simulink model "example_Hydraulic_HouseHeatingSystem"  (R2016b)
settings: Solver=ode23tb  StartTime=0.0  StopTime=2*24*3600  MaxStep=3600  RelTol=1e-3  EnableMultiTasking=on
undefined symbols (not defined in the file): path_carnot
libraries: carnot x12
settings Model: Creator=drhf  LastModifiedBy=drhf
settings DataIOCC: LimitDataPoints=on  SaveFormat=Array  SignalLoggingSaveFormat=ModelDataLogs
settings OptimizationCC: ExpressionDepthLimit=2147483647  LifeSpan=inf
settings DebuggingCC: UnderspecifiedInitializationDetection=Classic  MergeDetectMultiDrivingBlocksExec=none  SolverPrmCheckMsg=warning  FcnCallInpInsideContextMsg=warning  StateNameClashWarn=warning  SFUnexpectedBacktrackingDiag=warning  SFNoUnconditionalDefaultTransitionDiag=warning  SFExecutionAtInitializationDiag=none
settings HardwareCC: ProdBitPerPointer=32  ProdBitPerSizeT=32  ProdBitPerPtrDiffT=32  ProdLargestAtomicFloat=None  ProdIntDivRoundTo=Undefined  ProdEndianess=Unspecified  ProdWordSize=32  ProdHWDeviceType=32-bit Generic
settings ModelReferenceCC: PropagateSignalLabelsOutOfModel=off
settings GRTTargetCC: TargetLangStandard=C89/C90 (ANSI)  GeneratePreprocessorConditionals=Disable all  CombineOutputUpdateFcns=off  GRTInterface=on
settings ConfigComp: CovMetricSettings=dw  CovHtmlReporting=on  CovSaveCumulativeToWorkspaceVar=on  CovSaveSingleToWorkspaceVar=on  CovExternalEMLEnable=off

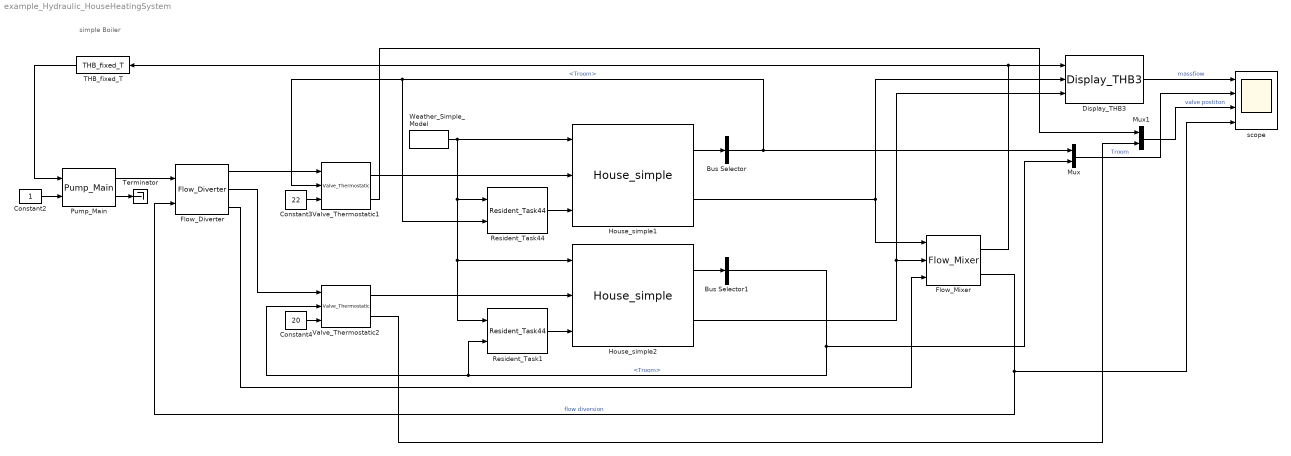
== system example_Hydraulic_HouseHeatingSystem ==
  note: simple Boiler
  Bus Selector : BusSelector  OutputSignals=Troom
  Bus Selector1 : BusSelector  OutputSignals=Troom
  Constant2 : Constant
  Constant3 : Constant  Value=22
  Constant4 : Constant  Value=20
  Display_THB3 : carnot/Outputs/Display_THB3  t=off  m=on  p=off  id=off  mix=off  d=off
  Flow_Diverter : carnot/Hydraulics/Flow_Diverter
  Flow_Mixer : carnot/Hydraulics/Flow_Mixer  t=1
  House_simple1 : carnot/Load/Houses/House_simple  tini=20  dtroom=inf  Tmeaninside=23.8  deltathetai=3.8  Tmeanoutside=11  deltathetae=9.3  tshift=319*3600  PathName=fullfile(path_carnot('libsl'), 'Load', 'Houses', 'House_simple', 'parameter_set')  FileName='SimpleHouse_Room40m2.mat'  userPath=off  userParam=off  Ahabit=40  Hroom=2.5  slabwidth=10  slablength=7  dwall=0.4  UAwall=100  capa=500000  utot=0.183  gammat=0  cond_ground=2  cp_ground=800  rho_ground=2500  Awindow=[12 4 3 4]  AziWin=[0 90 -180 -90]  Uwindow=[2 2 2 2]  Gwindow=[0.5 0.5 0.5 0.5]  alpha=10  H=1.2  W=1  Nwin=4  Ventilationrate=0.4  Heatrecovery=0  pnom=10000  dtnom=49.83  expo=1.3  mcap=10*4812  lin=100  qua=100
  House_simple2 : carnot/Load/Houses/House_simple  tini=20  dtroom=inf  Tmeaninside=23.8  deltathetai=3.8  Tmeanoutside=11  deltathetae=9.3  tshift=319*3600  PathName=fullfile(path_carnot('libsl'), 'Load', 'Houses', 'House_simple', 'parameter_set')  FileName='SimpleHouse_Room40m2.mat'  userPath=off  userParam=off  Ahabit=40  Hroom=2.5  slabwidth=10  slablength=7  dwall=0.4  UAwall=100  capa=500000  utot=0.183  gammat=0  cond_ground=2  cp_ground=800  rho_ground=2500  Awindow=[12 4 3 4]  AziWin=[0 90 -180 -90]  Uwindow=[2 2 2 2]  Gwindow=[0.5 0.5 0.5 0.5]  alpha=10  H=1.2  W=1  Nwin=4  Ventilationrate=0.4  Heatrecovery=0  pnom=10000  dtnom=49.83  expo=1.3  mcap=10*4812  lin=100  qua=100
  Mux : Mux  Inputs=2
  Mux1 : Mux  Inputs=2
  Pump_Main : carnot/Hydraulics/Pump_Main  Tini=20  p0=3e5  IDpreset=pressure drop  fluid=Water  mix=0  mix2=0  mix3=0  t1=1  PathName=fullfile(path_carnot('libsl'), 'Hydraulics', 'Pump_Main', 'parameter_set')  FileName='Pump6m.mat'  userPath=off  userParam=off  a0=60000  a1=-43200  a2=0  dia=0.025  UA=1  mcp=4182  e0=50  e1=28.8  e2=-10.368
  Resident_Task1 : carnot/Load/Houses/Resident_Task44  period=24*3600  rep_seq_te=[0 1 6 7 8 9 11 12 13 18 19 20 22 23]*3600  rep_seq_de=[1 5 1 1 1 2 1 1 4 2 1 2 1 1]*3600  rep_seq_ye=[105 55 392.5 457.5 420 55 250 55 120 170 615 420 442.5 355]/3  rep_seq_to=[0 6 7 8 9 11 12 13 14 15 17 18 20 21 22]*3600  rep_seq_do=[6 1 1 1 2 1 1 1 1 2 1 2 1 1 2]*3600  rep_seq_yo=[4 2 3 2 0 1 3 2 1 0 1 2 4 3 4]*60/2  Topen=24  Tclose=23  TrAboveTa=2  TaTooCold=12  timeFIR=24  TaIni=12  starttime=8  stoptime=22  TroomShadeOn=23.8  TroomShadeOff=22.8  SolarShadeOn=300  SolarShadeOff=200  max_shade=1  CalcAirComp=off  mdotCO2=0  mdotH2O=0  mdotVOC=0
  Resident_Task44 : carnot/Load/Houses/Resident_Task44  period=24*3600  rep_seq_te=[0 1 6 7 8 9 11 12 13 18 19 20 22 23]*3600  rep_seq_de=[1 5 1 1 1 2 1 1 4 2 1 2 1 1]*3600  rep_seq_ye=[105 55 392.5 457.5 420 55 250 55 120 170 615 420 442.5 355]/3  rep_seq_to=[0 6 7 8 9 11 12 13 14 15 17 18 20 21 22]*3600  rep_seq_do=[6 1 1 1 2 1 1 1 1 2 1 2 1 1 2]*3600  rep_seq_yo=[4 2 3 2 0 1 3 2 1 0 1 2 4 3 4]*60/2  Topen=24  Tclose=23  TrAboveTa=2  TaTooCold=12  timeFIR=24  TaIni=12  starttime=8  stoptime=22  TroomShadeOn=23.8  TroomShadeOff=22.8  SolarShadeOn=300  SolarShadeOff=200  max_shade=1  CalcAirComp=off  mdotCO2=0  mdotH2O=0  mdotVOC=0
  THB_fixed_T : carnot/Source/Simple/THB_fixed_T  t=60
  Terminator : Terminator
  Valve_Thermostatic1 : carnot/Hydraulics/Valve_Thermostatic  p=4  op=0.5  bl=0.1  ts=1  dt_V=1  ART=linear  kvs=2  psi_0=0.04
  Valve_Thermostatic2 : carnot/Hydraulics/Valve_Thermostatic  p=4  op=0.5  bl=0.1  ts=1  dt_V=1  ART=linear  kvs=2  psi_0=0.04
  Weather_Simple_Model : carnot/Weather/Weather_Simple_Model  lat=60  Ibn=0  Idg=0  tamb=-5  deltaTsky=-6  rh=50  precip="10e-3/24/3600           % 10 mm in 24 h"  cloud=0.125  p=1013e2  vw=1  wdir=270
  scope : Scope  NumInputPorts=4
  wires:
  Constant2/1 -> Pump_Main/2
  Pump_Main/2 -> Terminator/1
  Pump_Main/1 -> Flow_Diverter/1
  Flow_Diverter/1 -> Valve_Thermostatic1/1
  House_simple2/1 -> Bus Selector1/1
  Flow_Diverter/2 -> Valve_Thermostatic2/1
  Flow_Diverter/3 -> Flow_Mixer/3
  Flow_Mixer/2 -> Flow_Diverter/2, scope/4  "flow diversion"
  Flow_Mixer/1 -> THB_fixed_T/1, Display_THB3/1
  Display_THB3/1 -> scope/1  "massfiow"
  Mux1/1 -> scope/3  "valve postiton"
  House_simple2/2 -> Display_THB3/3, Flow_Mixer/2
  House_simple1/2 -> Display_THB3/2, Flow_Mixer/1
  Valve_Thermostatic1/2 -> Mux1/1
  Valve_Thermostatic2/2 -> Mux1/2
  Constant3/1 -> Valve_Thermostatic1/3
  Constant4/1 -> Valve_Thermostatic2/3
  Mux/1 -> scope/2  "Troom"
  Valve_Thermostatic1/1 -> House_simple1/2
  Weather_Simple_Model/1 -> House_simple1/1, Resident_Task44/1, Resident_Task1/1, House_simple2/1
  Valve_Thermostatic2/1 -> House_simple2/2
  THB_fixed_T/1 -> Pump_Main/1
  Bus Selector/1 -> Resident_Task44/2, Valve_Thermostatic1/2, Mux/1  "<Troom>"
  Bus Selector1/1 -> Resident_Task1/2, Valve_Thermostatic2/2, Mux/2  "<Troom>"
  House_simple1/1 -> Bus Selector/1
  Resident_Task44/1 -> House_simple1/3
  Resident_Task1/1 -> House_simple2/3
